simulink model "yaw_lin"  (R2017b)
settings: Solver=VariableStepAuto  StartTime=0.0  StopTime=10  RelTol=1e-3
values from neighbouring files (symbols this model uses):
  J = 0.0007    [Motor_Parameters.m]    (also in startup.m = 0.0008)
  wb = .6    (= 0.6)    [Quad_vis.m]    (also in Sim_Constants.m; startup.m)
undefined symbols (not defined in the file or in its folder): Izz
libraries: simulink x2, simulink_extras x2
settings Model: Creator=schapman  LastModifiedBy=DanAdmin

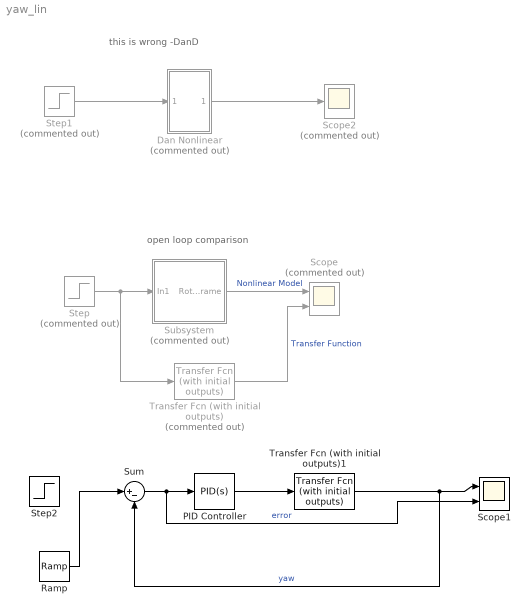
== system yaw_lin ==
  note: open loop comparison
  note: this is wrong -DanD
  Dan Nonlinear : Subsystem  Commented=on
  PID Controller : simulink/Continuous/PID Controller  Controller=PID  TimeDomain=Continuous-time  SampleTime=-1  IntegratorMethod=Forward Euler  FilterMethod=Forward Euler  Form=Parallel  UseFilter=on  ControllerParametersSource=internal  P=3969499.29287214  I=719645.642029045  D=5376455.39092611  N=21.1209167612032  InitialConditionSource=internal  InitialConditionForIntegrator=0  InitialConditionForFilter=0  ExternalReset=none  LimitOutput=off  UpperSaturationLimit=inf  LowerSaturationLimit=-inf  LinearizeAsGain=on  AntiWindupMode=none  Kb=1  TrackingMode=off  Kt=1  PParamMin=[]  PParamMax=[]  IParamMin=[]  IParamMax=[]  DParamMin=[]  DParamMax=[]  NParamMin=[]  NParamMax=[]  KbParamMin=[]  KbParamMax=[]  KtParamMin=[]  KtParamMax=[]  POutMin=[]  POutMax=[]  IOutMin=[]  IOutMax=[]  DOutMin=[]  DOutMax=[]  NOutMin=[]  NOutMax=[]  KbOutMin=[]  KbOutMax=[]  KtOutMin=[]  KtOutMax=[]  IntegratorOutMin=[]  IntegratorOutMax=[]  FilterOutMin=[]  FilterOutMax=[]  SumOutMin=[]  SumOutMax=[]  SumI1OutMin=[]  SumI1OutMax=[]  SumI2OutMin=[]  SumI2OutMax=[]  SumI3OutMin=[]  SumI3OutMax=[]  SumDOutMin=[]  SumDOutMax=[]  SaturationOutMin=[]  SaturationOutMax=[]  IntegratorContinuousStateAttributes=''  IntegratorStateMustResolveToSignalObject=off  IntegratorRTWStateStorageClass=Auto  FilterContinuousStateAttributes=''  FilterStateMustResolveToSignalObject=off  FilterRTWStateStorageClass=Auto  DifferentiatorICPrevScaledInput=0  DifferentiatorOutMin=[]  DifferentiatorOutMax=[]  InitialConditionSetting=State (most efficient)  FilterDiffOutCoefMin=[]  FilterDiffOutCoefMax=[]  SumDenOutMin=[]  SumDenOutMax=[]  SumNumOutMin=[]  SumNumOutMax=[]  ReciprocalOutMin=[]  ReciprocalOutMax=[]  DivideOutMin=[]  DivideOutMax=[]  TunerSelectOption=Transfer Function Based (PID Tuner App)
  Ramp : simulink/Sources/Ramp  slope=pi/4  start=0  X0=0
  Scope : Scope  Commented=on  NumInputPorts=2
  Scope1 : Scope  NumInputPorts=2
  Scope2 : Scope  Commented=on
  Step : Step  Commented=on  Time=2  After=10000  SampleTime=0
  Step1 : Step  Commented=on  Time=2  After=10000  SampleTime=0
  Step2 : Step  After=0.2  SampleTime=0
  Subsystem : Subsystem  Commented=on
  Sum : Sum  Inputs=|+-
  Transfer Fcn (with initial outputs) : simulink_extras/Additional Linear/Transfer Fcn (with initial outputs)  Commented=on  N=[7.015e-07]  D="[1  0 0]"  Y0=0  U0=0
  Transfer Fcn (with initial outputs)1 : simulink_extras/Additional Linear/Transfer Fcn (with initial outputs)  N=[7.015e-07]  D="[1  0 0]"  Y0=0  U0=0
  wires:
  Step/1 -> Transfer Fcn (with initial outputs)/1, Subsystem/1(In1)
  Subsystem/1(Rotation in BODY frame) -> Scope/1  "Nonlinear Model"
  Transfer Fcn (with initial outputs)1/1 -> Sum/2, Scope1/1  "yaw"
  Sum/1 -> Scope1/2, PID Controller/1  "error"
  Ramp/1 -> Sum/1
  PID Controller/1 -> Transfer Fcn (with initial outputs)1/1
  Transfer Fcn (with initial outputs)/1 -> Scope/2  "Transfer Function"
  Step1/1 -> Dan Nonlinear/1(In1)
  Dan Nonlinear/1(Yaw) -> Scope2/1

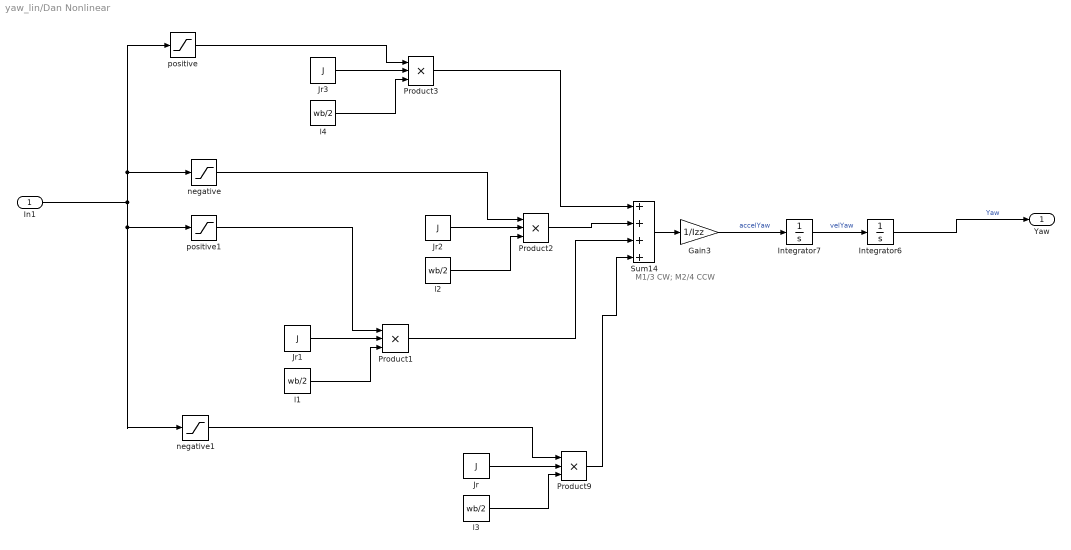
== system yaw_lin/Dan Nonlinear ==
  note: M1/3 CW; M2/4 CCW
  In1 : Inport
  Gain3 : Gain  Gain=1/Izz
  Integrator6 : Integrator
  Integrator7 : Integrator
  Jr{,1..3} (4 alike) : Constant  Value=J
  Product{1..3,9} (4 alike) : Product  Inputs=3
  Sum14 : Sum  Inputs=++++
  l{1..4} (4 alike) : Constant  Value=wb/2
  negative : Saturate  UpperLimit=0  LowerLimit=-inf
  negative1 : Saturate  UpperLimit=0  LowerLimit=-inf
  positive : Saturate  UpperLimit=inf  LowerLimit=0
  positive1 : Saturate  UpperLimit=inf  LowerLimit=0
  Yaw : Outport
  wires:
  Jr/1 -> Product9/2
  Integrator6/1 -> Yaw/1  "Yaw"
  Gain3/1 -> Integrator7/1  "accelYaw"
  Product9/1 -> Sum14/4
  Sum14/1 -> Gain3/1
  Integrator7/1 -> Integrator6/1  "velYaw"
  Product3/1 -> Sum14/1
  In1/1 -> positive1/1, negative1/1, positive/1, negative/1
  Product1/1 -> Sum14/3
  Product2/1 -> Sum14/2
  l3/1 -> Product9/3
  Jr1/1 -> Product1/2
  l1/1 -> Product1/3
  l2/1 -> Product2/3
  Jr2/1 -> Product2/2
  l4/1 -> Product3/3
  Jr3/1 -> Product3/2
  negative1/1 -> Product9/1
  negative/1 -> Product2/1
  positive/1 -> Product3/1
  positive1/1 -> Product1/1

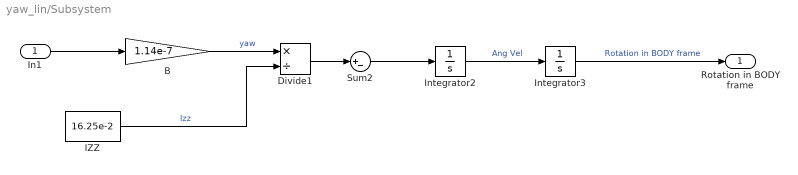
== system yaw_lin/Subsystem ==
  In1 : Inport
  B : Gain  Gain=1.14e-7
  Divide1 : Product  Inputs=*/
  IZZ : Constant  Value=16.25e-2
  Integrator2 : Integrator
  Integrator3 : Integrator
  Sum2 : Sum  Inputs=|+-
  Rotation in BODY frame : Outport
  wires:
  Integrator3/1 -> Rotation in BODY frame/1  "Rotation in BODY frame"
  IZZ/1 -> Divide1/2  "Izz"
  Integrator2/1 -> Integrator3/1  "Ang Vel"
  Divide1/1 -> Sum2/1
  B/1 -> Divide1/1  "yaw"
  Sum2/1 -> Integrator2/1
  In1/1 -> B/1
